simulink model "lab2_ali"  (R2024b)
settings: Solver=VariableStepAuto  StartTime=0.0  StopTime=5  RelTol=1e-4
values from neighbouring files (symbols this model uses):
  A0 = A22_prime-L*A12_prime    [code_ali.m]    (also in lab2_challenge_ali.m)
  AB = inv(eye(1) - A0*T_s)    [code_ali.m]    (also in lab2_challenge_ali.m)
  AF = REG_disc.A    [code_ali.m]    (also in lab2_challenge_ali.m)
  B0 = [B_prime(2)-L*B_prime(1),A0*L+A_prime(2,1)-L*A_prime(1,1)]    [code_ali.m]    (also in lab2_challenge_ali.m)
  BB = AB * B0 * T_s    [code_ali.m]    (also in lab2_challenge_ali.m)
  BF = REG_disc.B    [code_ali.m]    (also in lab2_challenge_ali.m)
  C0 = T_trsf*[0;1]    [code_ali.m]    (also in lab2_challenge_ali.m)
  CB = C0*AB    [code_ali.m]    (also in lab2_challenge_ali.m)
  CF = REG_disc.C    [code_ali.m]    (also in lab2_challenge_ali.m)
  D0 = T_trsf*[0,1;0,L]    [code_ali.m]    (also in lab2_challenge_ali.m)
  DB = D0 + C0*BB    [code_ali.m]    (also in lab2_challenge_ali.m)
  degs2rpm = 60/360    (= 0.166666666667)    [Init_ali.m]
  DF = REG_disc.D    [code_ali.m]    (also in lab2_challenge_ali.m)
  K = acker(A,B,poles)    [code_ali.m]    (also in lab2_challenge_ali.m)
  K2 = K_robust(2:3)    [code_ali.m]    (also in lab2_challenge_ali.m)
  KI = K_robust(1)    [code_ali.m]    (also in lab2_challenge_ali.m)
  Nu = Ans(3,1)    [code_ali.m]    (also in lab2_challenge_ali.m)
  Nx = Ans(1:2,1)    [code_ali.m]    (also in lab2_challenge_ali.m)
  rpm2rads = 2*pi/60    (= 0.10471975512)    [Init_ali.m]
  T_s = 0.001*10    (= 0.01)    [code_ali.m]    (also in lab2_challenge_ali.m)
undefined symbols (not defined in the file or in its folder): DiscIntNeverNeededParam
settings Model: Creator=riccardo  LastModifiedBy=Ali
settings SolverCC: AlgebraicLoopSolver=TrustRegion
settings DebuggingCC: UnconnectedInputMsg=warning  UnconnectedOutputMsg=warning  UnconnectedLineMsg=warning
settings ModelReferenceCC: EnableRefExpFcnMdlSchedulingChecks=on
settings RTWCC: GPUComputeCapability=3.5

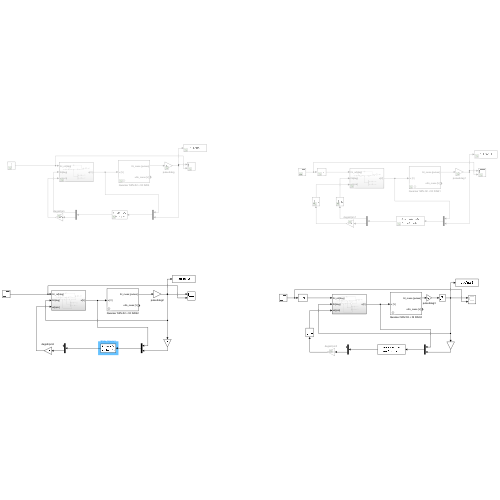
[thumbnail: Simulink's stored preview of the top-level diagram]
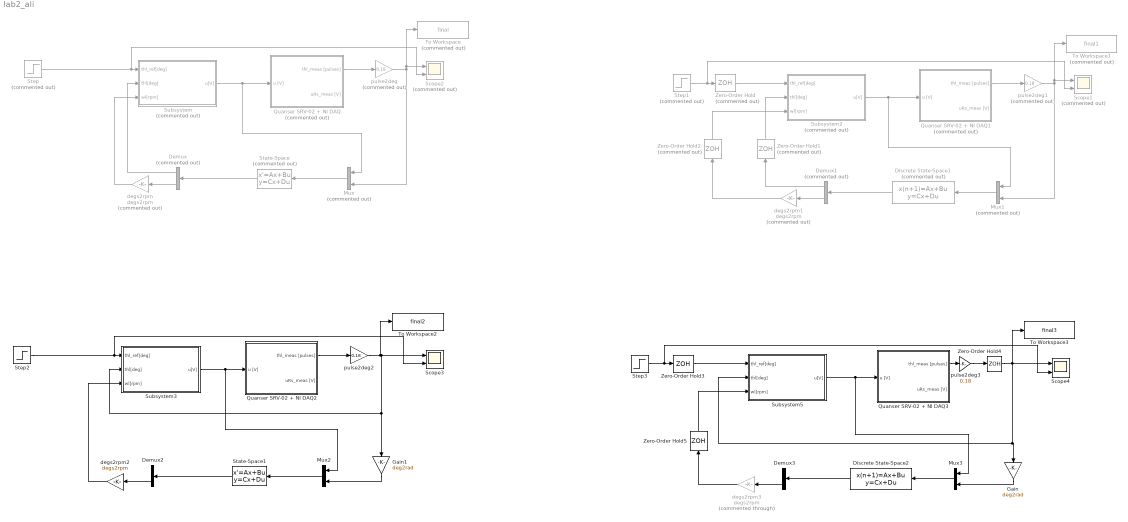
== system lab2_ali ==
  Demux : Demux  Commented=on  Outputs=2
  Demux1 : Demux  Commented=on  Outputs=2
  Demux2 : Demux  Outputs=2
  Demux3 : Demux  Outputs=2
  Discrete State-Space1 : DiscreteStateSpace  Commented=on  A=AF  B=BF  C=CF  D=DF  SampleTime=T_s
  Discrete State-Space2 : DiscreteStateSpace  A=AB  B=BB  C=CB  D=DB  SampleTime=T_s
  Gain : Gain  Gain=deg2rad
  Gain1 : Gain  Gain=deg2rad
  Mux : Mux  Commented=on  Inputs=2
  Mux1 : Mux  Commented=on  Inputs=2
  Mux2 : Mux  Inputs=2
  Mux3 : Mux  Inputs=2
  Quanser SRV-02 + NI DAQ : Subsystem  Commented=on  mask(Quanser SRV-02 (with inertial load) + NI DAQ){Ts=0.001, fricType=Coulomb + viscous}
      mask prompts: Ts "NI DAQ Sample Time:"; fricType "Friction model"
      mask help: Quanser SRV-02 (with inertial load) + NI DAQ model.
      mask init:
      | %%  Sensors data
      | 
      | %   shunt resistor
      | sens.curr.Rs = 0.5;                         %   resistance [Ohm]   
      | sens.curr.uRs_std = 0.01;                   %   voltage noise standard dev [V]                           
      | sens.curr.uRs_var = sens.curr.uRs_std^2;	%   voltage noise variance [V^2]
      | 
      | %   Hewlett-Packard HEDS-5540#A06 optical encoder
      | sens.enc.ppr = 500*4;                       %   pulses per rotation
      | sens.enc.pulse2deg = 360/sens.enc.ppr;      %   [pulses] -> [deg]
      | sens.enc.pulse2rad = 2*pi/sens.enc.ppr;     %   [pulses] -> [rad]
      | sens.enc.deg2pulse = sens.enc.ppr/360;      %   [deg] -> [pulses]
      | sens.enc.rad2pulse = sens.enc.ppr/2/pi;     %   [rad] -> [pulses]
      | 
      | 
      | %%  Data acquisition board (daq) data
      | 
      | %   NI PCI-6221 DAC data
      | daq.dac.bits = 16;                                  %   resolution (bits)
      | daq.dac.fs   = 10;                                  %   full scale 
      | daq.dac.q    = 2*daq.dac.fs/(2^daq.dac.bits-1);     %	quantization
      | 
      | %   NI PCI-6221 ADC data
      | daq.adc.bits = 16;                                  %   resolution (bits)
      | daq.adc.fs   = 10;                                  %   full scale (as set in SLDRT Analog Input block)
      | daq.adc.q    = 2*daq.adc.fs/(2^daq.adc.bits-1);     %   quantization
      mask Help:
      | Riccardo Antonello (antonello@dei.unipd.it)
      | 
      | April 24, 2020
      | 
      | Dept. of Information Engineering, University of Padova
      mask TypeOptions fricType: Coulomb + viscous | Karnopp
  Quanser SRV-02 + NI DAQ1 : Subsystem  Commented=on  mask(Quanser SRV-02 (with inertial load) + NI DAQ){Ts=T_s, fricType=Coulomb + viscous}
      mask prompts: Ts "NI DAQ Sample Time:"; fricType "Friction model"
      mask help: Quanser SRV-02 (with inertial load) + NI DAQ model.
      mask init: same as lab2_ali/Quanser SRV-02 + NI DAQ
      mask Help:
      | Riccardo Antonello (antonello@dei.unipd.it)
      | 
      | April 24, 2020
      | 
      | Dept. of Information Engineering, University of Padova
      mask TypeOptions fricType: Coulomb + viscous | Karnopp
  Quanser SRV-02 + NI DAQ2 : Subsystem  mask(Quanser SRV-02 (with inertial load) + NI DAQ){Ts=0.001, fricType=Coulomb + viscous}
      mask prompts: Ts "NI DAQ Sample Time:"; fricType "Friction model"
      mask help: Quanser SRV-02 (with inertial load) + NI DAQ model.
      mask init: same as lab2_ali/Quanser SRV-02 + NI DAQ
      mask Help:
      | Riccardo Antonello (antonello@dei.unipd.it)
      | 
      | April 24, 2020
      | 
      | Dept. of Information Engineering, University of Padova
      mask TypeOptions fricType: Coulomb + viscous | Karnopp
  Quanser SRV-02 + NI DAQ3 : Subsystem  mask(Quanser SRV-02 (with inertial load) + NI DAQ){Ts=T_s, fricType=Coulomb + viscous}
      mask prompts: Ts "NI DAQ Sample Time:"; fricType "Friction model"
      mask help: Quanser SRV-02 (with inertial load) + NI DAQ model.
      mask init: same as lab2_ali/Quanser SRV-02 + NI DAQ
      mask Help:
      | Riccardo Antonello (antonello@dei.unipd.it)
      | 
      | April 24, 2020
      | 
      | Dept. of Information Engineering, University of Padova
      mask TypeOptions fricType: Coulomb + viscous | Karnopp
  Scope1 : Scope  Commented=on  NumInputPorts=2
  Scope2 : Scope  Commented=on  NumInputPorts=2
  Scope3 : Scope  NumInputPorts=2
  Scope4 : Scope  NumInputPorts=2
  State-Space : StateSpace  Commented=on  A=A0  B=B0  C=C0  D=D0  InitialCondition=0
  State-Space1 : StateSpace  A=A0  B=B0  C=C0  D=D0  InitialCondition=0
  Step : Step  Commented=on  Time=0  After=40  SampleTime=0
  Step1 : Step  Commented=on  Time=0  After=50  SampleTime=T_s
  Step2 : Step  Time=0  After=60  SampleTime=0
  Step3 : Step  Time=0  After=60  SampleTime=T_s
  Subsystem : Subsystem  Commented=on
  Subsystem2 : Subsystem  Commented=on
  Subsystem3 : Subsystem
  Subsystem5 : Subsystem
  To Workspace : ToWorkspace  Commented=on  VariableName=final  SaveFormat=Structure With Time  SampleTime=-1
  To Workspace1 : ToWorkspace  Commented=on  VariableName=final1  SaveFormat=Structure With Time  SampleTime=-1
  To Workspace2 : ToWorkspace  VariableName=final2  SaveFormat=Structure With Time  SampleTime=-1
  To Workspace3 : ToWorkspace  VariableName=final3  SaveFormat=Structure With Time  SampleTime=-1
  Zero-Order Hold : ZeroOrderHold  Commented=on  SampleTime=T_s
  Zero-Order Hold1 : ZeroOrderHold  Commented=on  SampleTime=T_s
  Zero-Order Hold2 : ZeroOrderHold  Commented=on  SampleTime=T_s
  Zero-Order Hold3 : ZeroOrderHold  SampleTime=T_s
  Zero-Order Hold4 : ZeroOrderHold  SampleTime=T_s
  Zero-Order Hold5 : ZeroOrderHold  SampleTime=T_s
  degs2rpm : Gain  Commented=on  Gain=degs2rpm
  degs2rpm1 : Gain  Commented=on  Gain=degs2rpm
  degs2rpm2 : Gain  Gain=degs2rpm
  degs2rpm3 : Gain  Commented=through  Gain=degs2rpm
  pulse2deg : Gain  Commented=on  Gain=0.18
  pulse2deg1 : Gain  Commented=on  Gain=0.18
  pulse2deg2 : Gain  Gain=0.18
  pulse2deg3 : Gain  Gain=0.18
  wires:
  Step/1 -> Scope2/2, Subsystem/1(thl_ref[deg])
  Quanser SRV-02 + NI DAQ/1(thl_meas [pulses]) -> pulse2deg/1
  pulse2deg/1 -> To Workspace/1, Scope2/1, Mux/2
  Mux/1 -> State-Space/1
  Subsystem/1(u[V]) -> Quanser SRV-02 + NI DAQ/1(u [V]), Mux/1
  State-Space/1 -> Demux/1
  Demux/2 -> degs2rpm/1
  degs2rpm/1 -> Subsystem/3(wl[rpm])
  Demux/1 -> Subsystem/2(thl[deg])
  Mux1/1 -> Discrete State-Space1/1
  Subsystem2/1(u[V]) -> Quanser SRV-02 + NI DAQ1/1(u [V]), Mux1/1
  pulse2deg1/1 -> To Workspace1/1, Scope1/1, Mux1/2
  Step1/1 -> Scope1/2, Zero-Order Hold/1
  Demux1/2 -> degs2rpm1/1
  Discrete State-Space1/1 -> Demux1/1
  degs2rpm1/1 -> Zero-Order Hold2/1
  Demux1/1 -> Zero-Order Hold1/1
  Quanser SRV-02 + NI DAQ1/1(thl_meas [pulses]) -> pulse2deg1/1
  Mux2/1 -> State-Space1/1
  Subsystem3/1(u[V]) -> Quanser SRV-02 + NI DAQ2/1(u [V]), Mux2/1
  pulse2deg2/1 -> Scope3/1, Subsystem3/2(thl[deg]), Gain1/1, To Workspace2/1
  Step2/1 -> Scope3/2, Subsystem3/1(thl_ref[deg])
  Demux2/2 -> degs2rpm2/1
  State-Space1/1 -> Demux2/1
  degs2rpm2/1 -> Subsystem3/3(wl[rpm])
  Quanser SRV-02 + NI DAQ2/1(thl_meas [pulses]) -> pulse2deg2/1
  Zero-Order Hold/1 -> Subsystem2/1(thl_ref[deg])
  Zero-Order Hold2/1 -> Subsystem2/3(wl[rpm])
  Zero-Order Hold1/1 -> Subsystem2/2(thl[deg])
  degs2rpm3/1 -> Zero-Order Hold5/1
  Step3/1 -> Scope4/2, Zero-Order Hold3/1
  Quanser SRV-02 + NI DAQ3/1(thl_meas [pulses]) -> pulse2deg3/1
  Demux3/2 -> degs2rpm3/1
  Discrete State-Space2/1 -> Demux3/1
  Subsystem5/1(u[V]) -> Quanser SRV-02 + NI DAQ3/1(u [V]), Mux3/1
  Mux3/1 -> Discrete State-Space2/1
  Zero-Order Hold3/1 -> Subsystem5/1(thl_ref[deg])
  pulse2deg3/1 -> Zero-Order Hold4/1
  Zero-Order Hold5/1 -> Subsystem5/3(wl[rpm])
  Gain/1 -> Mux3/2
  Gain1/1 -> Mux2/2
  Zero-Order Hold4/1 -> To Workspace3/1, Scope4/1, Subsystem5/2(thl[deg]), Gain/1

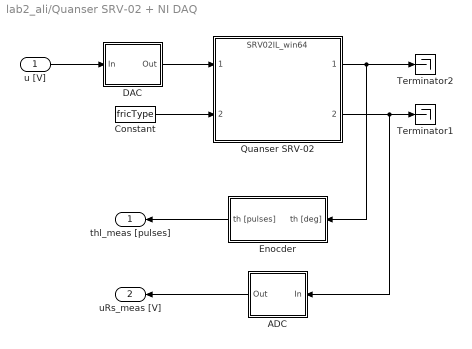
== system lab2_ali/Quanser SRV-02 + NI DAQ ==
  u [V] : Inport
  ADC : Subsystem
  Constant : Constant  Value=fricType
  DAC : Subsystem
  Enocder : Subsystem
  Quanser SRV-02 : ModelReference  ModelNameDialog=SRV02IL_win64.slxp  ModelReferenceVersion=1.44  CopyOfModelProtected=on
  Terminator1 : Terminator
  Terminator2 : Terminator
  thl_meas [pulses] : Outport
  uRs_meas [V] : Outport  Port=2
  wires:
  Enocder/1(th [pulses]) -> thl_meas [pulses]/1
  ADC/1(Out) -> uRs_meas [V]/1
  DAC/1(Out) -> Quanser SRV-02/1
  Quanser SRV-02/2 -> ADC/1(In), Terminator1/1
  u [V]/1 -> DAC/1(In)
  Quanser SRV-02/1 -> Enocder/1(th [deg]), Terminator2/1
  Constant/1 -> Quanser SRV-02/2

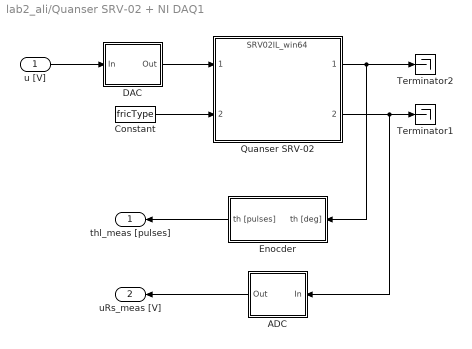
== system lab2_ali/Quanser SRV-02 + NI DAQ1 ==
  u [V] : Inport
  ADC : Subsystem
  Constant : Constant  Value=fricType
  DAC : Subsystem
  Enocder : Subsystem
  Quanser SRV-02 : ModelReference  ModelNameDialog=SRV02IL_win64.slxp  ModelReferenceVersion=1.44  CopyOfModelProtected=on
  Terminator1 : Terminator
  Terminator2 : Terminator
  thl_meas [pulses] : Outport
  uRs_meas [V] : Outport  Port=2
  wires:
  Enocder/1(th [pulses]) -> thl_meas [pulses]/1
  ADC/1(Out) -> uRs_meas [V]/1
  DAC/1(Out) -> Quanser SRV-02/1
  Quanser SRV-02/2 -> ADC/1(In), Terminator1/1
  u [V]/1 -> DAC/1(In)
  Quanser SRV-02/1 -> Enocder/1(th [deg]), Terminator2/1
  Constant/1 -> Quanser SRV-02/2

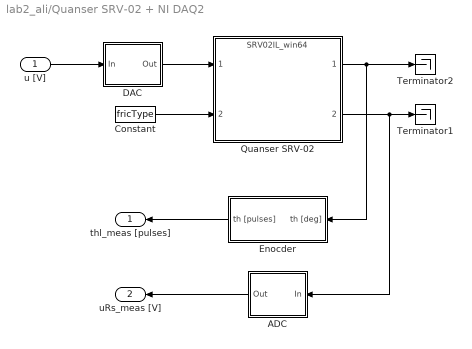
== system lab2_ali/Quanser SRV-02 + NI DAQ2 ==
  u [V] : Inport
  ADC : Subsystem
  Constant : Constant  Value=fricType
  DAC : Subsystem
  Enocder : Subsystem
  Quanser SRV-02 : ModelReference  ModelNameDialog=SRV02IL_win64.slxp  ModelReferenceVersion=1.44  CopyOfModelProtected=on
  Terminator1 : Terminator
  Terminator2 : Terminator
  thl_meas [pulses] : Outport
  uRs_meas [V] : Outport  Port=2
  wires:
  Enocder/1(th [pulses]) -> thl_meas [pulses]/1
  ADC/1(Out) -> uRs_meas [V]/1
  DAC/1(Out) -> Quanser SRV-02/1
  Quanser SRV-02/2 -> ADC/1(In), Terminator1/1
  u [V]/1 -> DAC/1(In)
  Quanser SRV-02/1 -> Enocder/1(th [deg]), Terminator2/1
  Constant/1 -> Quanser SRV-02/2

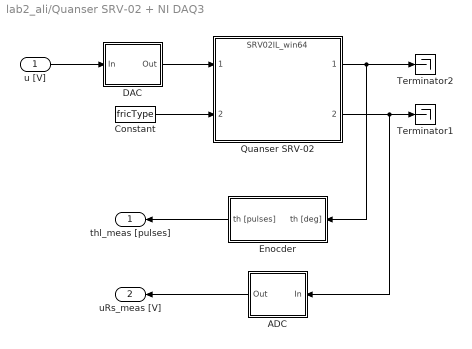
== system lab2_ali/Quanser SRV-02 + NI DAQ3 ==
  u [V] : Inport
  ADC : Subsystem
  Constant : Constant  Value=fricType
  DAC : Subsystem
  Enocder : Subsystem
  Quanser SRV-02 : ModelReference  ModelNameDialog=SRV02IL_win64.slxp  ModelReferenceVersion=1.44  CopyOfModelProtected=on
  Terminator1 : Terminator
  Terminator2 : Terminator
  thl_meas [pulses] : Outport
  uRs_meas [V] : Outport  Port=2
  wires:
  Enocder/1(th [pulses]) -> thl_meas [pulses]/1
  ADC/1(Out) -> uRs_meas [V]/1
  DAC/1(Out) -> Quanser SRV-02/1
  Quanser SRV-02/2 -> ADC/1(In), Terminator1/1
  u [V]/1 -> DAC/1(In)
  Quanser SRV-02/1 -> Enocder/1(th [deg]), Terminator2/1
  Constant/1 -> Quanser SRV-02/2

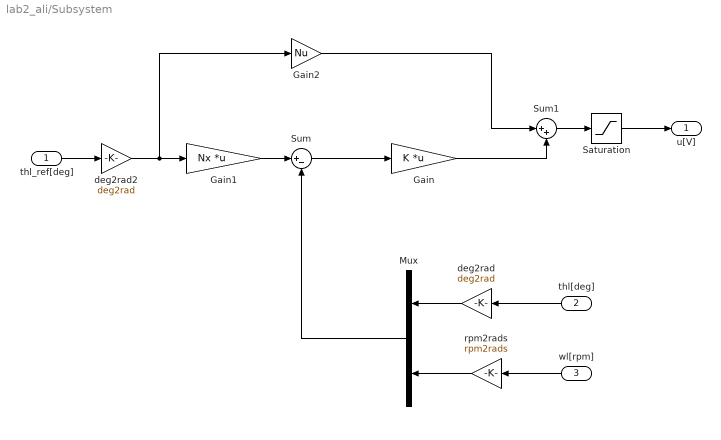
== system lab2_ali/Subsystem ==
  thl_ref[deg] : Inport
  thl[deg] : Inport  Port=2
  wl[rpm] : Inport  Port=3
  Gain : Gain  Gain=K  Multiplication=Matrix(K*u)
  Gain1 : Gain  Gain=Nx  Multiplication=Matrix(K*u)
  Gain2 : Gain  Gain=Nu
  Mux : Mux  Inputs=2
  Saturation : Saturate  UpperLimit=12  LowerLimit=-12
  Sum : Sum  Inputs=|+-
  Sum1 : Sum  Inputs=|++
  deg2rad : Gain  Gain=deg2rad
  deg2rad2 : Gain  Gain=deg2rad
  rpm2rads : Gain  Gain=rpm2rads
  u[V] : Outport
  wires:
  thl[deg]/1 -> deg2rad/1
  wl[rpm]/1 -> rpm2rads/1
  deg2rad/1 -> Mux/1
  rpm2rads/1 -> Mux/2
  Sum/1 -> Gain/1
  Gain1/1 -> Sum/1
  thl_ref[deg]/1 -> deg2rad2/1
  deg2rad2/1 -> Gain1/1, Gain2/1
  Gain2/1 -> Sum1/1
  Gain/1 -> Sum1/2
  Sum1/1 -> Saturation/1
  Saturation/1 -> u[V]/1
  Mux/1 -> Sum/2

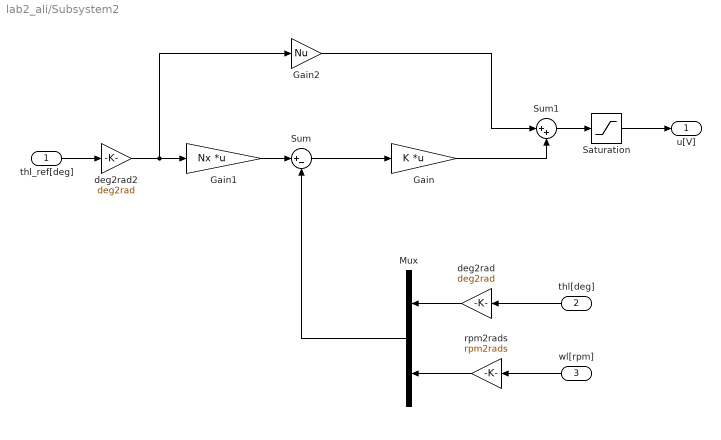
== system lab2_ali/Subsystem2 ==
  thl_ref[deg] : Inport
  thl[deg] : Inport  Port=2
  wl[rpm] : Inport  Port=3
  Gain : Gain  Gain=K  Multiplication=Matrix(K*u)
  Gain1 : Gain  Gain=Nx  Multiplication=Matrix(K*u)
  Gain2 : Gain  Gain=Nu
  Mux : Mux  Inputs=2
  Saturation : Saturate  UpperLimit=12  LowerLimit=-12
  Sum : Sum  Inputs=|+-
  Sum1 : Sum  Inputs=|++
  deg2rad : Gain  Gain=deg2rad
  deg2rad2 : Gain  Gain=deg2rad
  rpm2rads : Gain  Gain=rpm2rads
  u[V] : Outport
  wires:
  thl[deg]/1 -> deg2rad/1
  wl[rpm]/1 -> rpm2rads/1
  deg2rad/1 -> Mux/1
  rpm2rads/1 -> Mux/2
  Sum/1 -> Gain/1
  Gain1/1 -> Sum/1
  thl_ref[deg]/1 -> deg2rad2/1
  deg2rad2/1 -> Gain1/1, Gain2/1
  Gain2/1 -> Sum1/1
  Gain/1 -> Sum1/2
  Sum1/1 -> Saturation/1
  Saturation/1 -> u[V]/1
  Mux/1 -> Sum/2

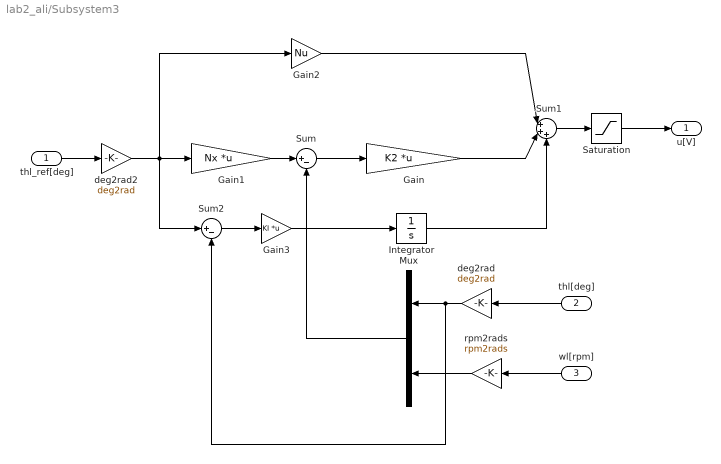
== system lab2_ali/Subsystem3 ==
  thl_ref[deg] : Inport
  thl[deg] : Inport  Port=2
  wl[rpm] : Inport  Port=3
  Gain : Gain  Gain=K2  Multiplication=Matrix(K*u)
  Gain1 : Gain  Gain=Nx  Multiplication=Matrix(K*u)
  Gain2 : Gain  Gain=Nu
  Gain3 : Gain  Gain=KI  Multiplication=Matrix(K*u)
  Integrator : Integrator
  Mux : Mux  Inputs=2
  Saturation : Saturate  UpperLimit=12  LowerLimit=-12
  Sum : Sum  Inputs=|+-
  Sum1 : Sum  Inputs=|+++
  Sum2 : Sum  Inputs=|+-
  deg2rad : Gain  Gain=deg2rad
  deg2rad2 : Gain  Gain=deg2rad
  rpm2rads : Gain  Gain=rpm2rads
  u[V] : Outport
  wires:
  thl[deg]/1 -> deg2rad/1
  wl[rpm]/1 -> rpm2rads/1
  deg2rad/1 -> Mux/1, Sum2/2
  rpm2rads/1 -> Mux/2
  Sum/1 -> Gain/1
  Gain1/1 -> Sum/1
  thl_ref[deg]/1 -> deg2rad2/1
  deg2rad2/1 -> Gain1/1, Sum2/1, Gain2/1
  Gain2/1 -> Sum1/1
  Gain/1 -> Sum1/2
  Sum1/1 -> Saturation/1
  Saturation/1 -> u[V]/1
  Integrator/1 -> Sum1/3
  Sum2/1 -> Gain3/1
  Gain3/1 -> Integrator/1
  Mux/1 -> Sum/2

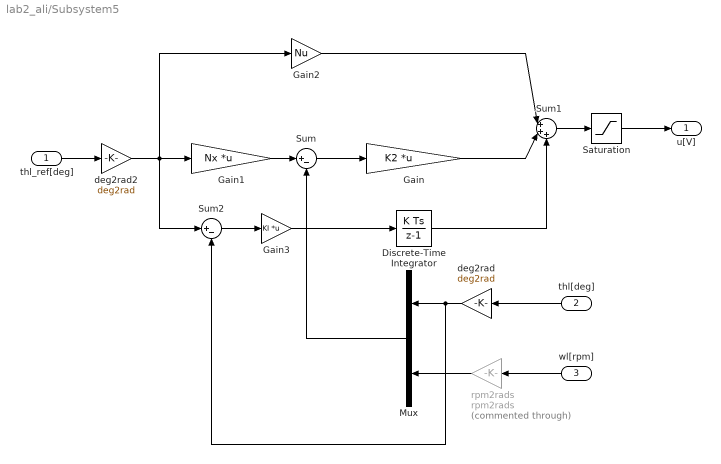
== system lab2_ali/Subsystem5 ==
  thl_ref[deg] : Inport
  thl[deg] : Inport  Port=2
  wl[rpm] : Inport  Port=3
  Discrete-Time Integrator : DiscreteIntegrator  gainval=1  SampleTime=T_s  ICPrevOutput=DiscIntNeverNeededParam  ICPrevScaledInput=DiscIntNeverNeededParam
  Gain : Gain  Gain=K2  Multiplication=Matrix(K*u)
  Gain1 : Gain  Gain=Nx  Multiplication=Matrix(K*u)
  Gain2 : Gain  Gain=Nu
  Gain3 : Gain  Gain=KI  Multiplication=Matrix(K*u)
  Mux : Mux  Inputs=2
  Saturation : Saturate  UpperLimit=12  LowerLimit=-12
  Sum : Sum  Inputs=|+-
  Sum1 : Sum  Inputs=|+++
  Sum2 : Sum  Inputs=|+-
  deg2rad : Gain  Gain=deg2rad
  deg2rad2 : Gain  Gain=deg2rad
  rpm2rads : Gain  Commented=through  Gain=rpm2rads
  u[V] : Outport
  wires:
  thl[deg]/1 -> deg2rad/1
  wl[rpm]/1 -> rpm2rads/1
  deg2rad/1 -> Mux/1, Sum2/2
  rpm2rads/1 -> Mux/2
  Sum/1 -> Gain/1
  Gain1/1 -> Sum/1
  thl_ref[deg]/1 -> deg2rad2/1
  deg2rad2/1 -> Gain1/1, Sum2/1, Gain2/1
  Gain2/1 -> Sum1/1
  Gain/1 -> Sum1/2
  Sum1/1 -> Saturation/1
  Saturation/1 -> u[V]/1
  Sum2/1 -> Gain3/1
  Gain3/1 -> Discrete-Time Integrator/1
  Mux/1 -> Sum/2
  Discrete-Time Integrator/1 -> Sum1/3

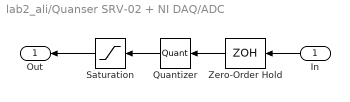
== system lab2_ali/Quanser SRV-02 + NI DAQ/ADC ==
  In : Inport
  Quantizer : Quantizer  QuantizationInterval=daq.adc.q
  Saturation : Saturate  UpperLimit=daq.adc.fs  LowerLimit=-daq.adc.fs
  Zero-Order Hold : ZeroOrderHold  SampleTime=Ts
  Out : Outport
  wires:
  Saturation/1 -> Out/1
  In/1 -> Zero-Order Hold/1
  Quantizer/1 -> Saturation/1
  Zero-Order Hold/1 -> Quantizer/1

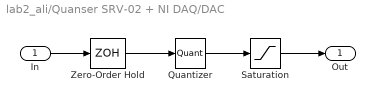
== system lab2_ali/Quanser SRV-02 + NI DAQ/DAC ==
  In : Inport
  Quantizer : Quantizer  QuantizationInterval=daq.dac.q
  Saturation : Saturate  UpperLimit=daq.dac.fs  LowerLimit=-daq.dac.fs
  Zero-Order Hold : ZeroOrderHold  SampleTime=Ts
  Out : Outport
  wires:
  Quantizer/1 -> Saturation/1
  In/1 -> Zero-Order Hold/1
  Zero-Order Hold/1 -> Quantizer/1
  Saturation/1 -> Out/1

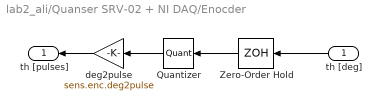
== system lab2_ali/Quanser SRV-02 + NI DAQ/Enocder ==
  th [deg] : Inport
  Quantizer : Quantizer  QuantizationInterval=sens.enc.pulse2deg
  Zero-Order Hold : ZeroOrderHold  SampleTime=Ts
  deg2pulse : Gain  Gain=sens.enc.deg2pulse
  th [pulses] : Outport
  wires:
  Quantizer/1 -> deg2pulse/1
  th [deg]/1 -> Zero-Order Hold/1
  Zero-Order Hold/1 -> Quantizer/1
  deg2pulse/1 -> th [pulses]/1

== system lab2_ali/Quanser SRV-02 + NI DAQ1/ADC ==
  In : Inport
  Quantizer : Quantizer  QuantizationInterval=daq.adc.q
  Saturation : Saturate  UpperLimit=daq.adc.fs  LowerLimit=-daq.adc.fs
  Zero-Order Hold : ZeroOrderHold  SampleTime=Ts
  Out : Outport
  wires:
  Saturation/1 -> Out/1
  In/1 -> Zero-Order Hold/1
  Quantizer/1 -> Saturation/1
  Zero-Order Hold/1 -> Quantizer/1

== system lab2_ali/Quanser SRV-02 + NI DAQ1/DAC ==
  In : Inport
  Quantizer : Quantizer  QuantizationInterval=daq.dac.q
  Saturation : Saturate  UpperLimit=daq.dac.fs  LowerLimit=-daq.dac.fs
  Zero-Order Hold : ZeroOrderHold  SampleTime=Ts
  Out : Outport
  wires:
  Quantizer/1 -> Saturation/1
  In/1 -> Zero-Order Hold/1
  Zero-Order Hold/1 -> Quantizer/1
  Saturation/1 -> Out/1

== system lab2_ali/Quanser SRV-02 + NI DAQ1/Enocder ==
  th [deg] : Inport
  Quantizer : Quantizer  QuantizationInterval=sens.enc.pulse2deg
  Zero-Order Hold : ZeroOrderHold  SampleTime=Ts
  deg2pulse : Gain  Gain=sens.enc.deg2pulse
  th [pulses] : Outport
  wires:
  Quantizer/1 -> deg2pulse/1
  th [deg]/1 -> Zero-Order Hold/1
  Zero-Order Hold/1 -> Quantizer/1
  deg2pulse/1 -> th [pulses]/1

== system lab2_ali/Quanser SRV-02 + NI DAQ2/ADC ==
  In : Inport
  Quantizer : Quantizer  QuantizationInterval=daq.adc.q
  Saturation : Saturate  UpperLimit=daq.adc.fs  LowerLimit=-daq.adc.fs
  Zero-Order Hold : ZeroOrderHold  SampleTime=Ts
  Out : Outport
  wires:
  Saturation/1 -> Out/1
  In/1 -> Zero-Order Hold/1
  Quantizer/1 -> Saturation/1
  Zero-Order Hold/1 -> Quantizer/1

== system lab2_ali/Quanser SRV-02 + NI DAQ2/DAC ==
  In : Inport
  Quantizer : Quantizer  QuantizationInterval=daq.dac.q
  Saturation : Saturate  UpperLimit=daq.dac.fs  LowerLimit=-daq.dac.fs
  Zero-Order Hold : ZeroOrderHold  SampleTime=Ts
  Out : Outport
  wires:
  Quantizer/1 -> Saturation/1
  In/1 -> Zero-Order Hold/1
  Zero-Order Hold/1 -> Quantizer/1
  Saturation/1 -> Out/1

== system lab2_ali/Quanser SRV-02 + NI DAQ2/Enocder ==
  th [deg] : Inport
  Quantizer : Quantizer  QuantizationInterval=sens.enc.pulse2deg
  Zero-Order Hold : ZeroOrderHold  SampleTime=Ts
  deg2pulse : Gain  Gain=sens.enc.deg2pulse
  th [pulses] : Outport
  wires:
  Quantizer/1 -> deg2pulse/1
  th [deg]/1 -> Zero-Order Hold/1
  Zero-Order Hold/1 -> Quantizer/1
  deg2pulse/1 -> th [pulses]/1

== system lab2_ali/Quanser SRV-02 + NI DAQ3/ADC ==
  In : Inport
  Quantizer : Quantizer  QuantizationInterval=daq.adc.q
  Saturation : Saturate  UpperLimit=daq.adc.fs  LowerLimit=-daq.adc.fs
  Zero-Order Hold : ZeroOrderHold  SampleTime=Ts
  Out : Outport
  wires:
  Saturation/1 -> Out/1
  In/1 -> Zero-Order Hold/1
  Quantizer/1 -> Saturation/1
  Zero-Order Hold/1 -> Quantizer/1

== system lab2_ali/Quanser SRV-02 + NI DAQ3/DAC ==
  In : Inport
  Quantizer : Quantizer  QuantizationInterval=daq.dac.q
  Saturation : Saturate  UpperLimit=daq.dac.fs  LowerLimit=-daq.dac.fs
  Zero-Order Hold : ZeroOrderHold  SampleTime=Ts
  Out : Outport
  wires:
  Quantizer/1 -> Saturation/1
  In/1 -> Zero-Order Hold/1
  Zero-Order Hold/1 -> Quantizer/1
  Saturation/1 -> Out/1

== system lab2_ali/Quanser SRV-02 + NI DAQ3/Enocder ==
  th [deg] : Inport
  Quantizer : Quantizer  QuantizationInterval=sens.enc.pulse2deg
  Zero-Order Hold : ZeroOrderHold  SampleTime=Ts
  deg2pulse : Gain  Gain=sens.enc.deg2pulse
  th [pulses] : Outport
  wires:
  Quantizer/1 -> deg2pulse/1
  th [deg]/1 -> Zero-Order Hold/1
  Zero-Order Hold/1 -> Quantizer/1
  deg2pulse/1 -> th [pulses]/1
